simulink model "NeuronalNetwork"  (R2019b)
settings: Solver=VariableStepAuto  StartTime=0.0  StopTime=10.0  RelTol=1e-3
libraries: neural x1006
(part 3 of 11)

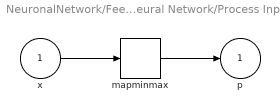
== system NeuronalNetwork/Feed-Forward Neural Network/Process Input 1 ==
  x : Inport  PortDimensions=1001  SampleTime=0.1
      mask Display: e = 0.06;c1 = [120 230 180]/255;c2 = ([120 230 180]+0)/(256+128);c3 = ([120 230 180]+128)/(256+128);patch([0 1 1 0],[0 0 1 1],c1);patch([0 1 1 1-e 1-e 0+e],[0 0 1 1-e 0+e 0+e],c2);patch([0 0 1 1-e 0+e 0+e],[0 1 1 1-e 1-e 0+e],c3);plot([0 1 1 0 0],[0 0 1 1 0]);
  mapminmax : neural/Processing Functions/mapminmax  xmin=[0.785398163397448278999490867136;0.709441408668645134838470767136;0.654230142742192599669692754105;0.615290765915770587746180808608;0.587466151596020225156280503143;0.565842136942244167130411369726;0.546291593455738633267060322396;0.525717673015665631908177601872;0.502090498167535370654945836577;0.474356865564650509448085813347;0.442284345023452152290133199131;0.406280540041972670906034181826;0.367209347491981086264445366396;0.326214334745977607710187839984;0.284555939084002673666873306502;0.243470447246644017269545656745;0.204059640191000424280787228781;0.167217606121480955039260152262;0.133595803186941530782405607169;0.10360143396444709829040675686;0.0774200746013615770380056346767;0.0550523483133633639852178021101;0.0363557636519837856781123264227;0.0210854164112119768503816885641;0.00892993062022617856143824610626;-0.000458871247863035236491668911185;-0.00744270835532989671889936289517;-0.0123794028861010652065033355029;-0.015610386427028499767288849398;-0.0174522405278876302503476836137;-0.0181914442101640538851370365592;-0.0180816228653828403594161500223;-0.0173427132861856403422962102923;-0.0161615638120036209102181601338;-0.014693574671496234529399771418;-0.0130650544686303771158009112696;-0.011376028220230871568219299661;-0.00970328347784943368026233656565;-0.00810348577435582306804917607224;-0.00661623389916599080606829375029;-0.00526695972456092675884065101855;-0.00406960663466815475430848891847;-0.00302904517984270427177762030624;-0.0021432046089739920091687963577;-0.00140491475077597627318937156815;-0.000803464748226234704020498611499;-0.00032589388241399674939202668611;4.19643425959570492977945832536e-05;0.000314660051512039018462019157596;0.000506500199471515699656265496742;0.000631090187944938207920131389983;0.000701017687264604560937186761294;0.000727653958252361121594731230289;0.000721049983764654456308562657796;0.000689907050786198183800479455385;0.000641603900344955846435368584935;0.000582265058452824391110880242195;0.000516857380913116060128231765702;0.000449304119792381939646475075278;0.000382607903842702157248822913971;0.000318975892022121954028079926502;0.00025994199600432033037122891983;0.000206482473331437432761958916672;0.000159122375285702943870091985445;0.000118031306518329159871427691542;8.31077348832920392851519864053e-05;5.4051700136836799970296851825e-05;3.04262305537150723466766066849e-05;1.17081084609615970748563995585e-05;-2.67115014418450869015941862017e-06;-1.32931011052050962462089955807e-05;-2.07278972408353467926644952968e-05;-2.5516458101115802037384128198e-05;-2.81582413605985237836648593657e-05;-2.91036346533601886221731547266e-05;-2.87500683957553349046065704897e-05;-2.7441043791043284727493301034e-05;-2.5467369312748289189585193526e-05;-2.30699985457327727544907247648e-05;-2.04439585727023143135738791898e-05;-1.77429484629065825629368191585e-05;-1.50842700734621359970333287492e-05;-1.25538272714997845014295307919e-05;-1.02109943727057839168992359191e-05;-8.09321005279528549181122798473e-06;-6.22019955787145306658203480765e-06;-4.5977662959106879725368344225e-06;-3.22112454465006692316819680855e-06;-2.07776889160626865304948296398e-06;-1.14989399091491861781832994893e-06;-4.16391101376589745086675975472e-07;1.45543456175900587368232663721e-07;5.59147637080315007551689632237e-07;8.47138112325396264168375637382e-07;1.03101689918894123820791719481e-06;1.13059865269882209304341813549e-06;1.16371964531403193632286274806e-06;1.1460927618056615528985275887e-06;1.09127662106800471519818529487e-06;1.01073089342484934149979380891e-06;9.13933864143956498082843609154e-07;8.08542119923316704444005154073e-07;7.00575833345595810897066257894e-07;5.94616389681945634038129355758e-07;4.94006026530158237619616556913e-07;4.01041718500749766462831757963e-07;3.17157717200089450670930091292e-07;2.43092999285821065313939470798e-07;1.79041373282728955018683336675e-07;1.24783202215539290591550525278e-07;7.97986305922648853083956055343e-08;4.33629090412779305552248843014e-08 ...(+32708 chars)]  xmax=[2.82842712474619029094924371748;2.6907248094147417916133235849;2.58020759331951055060017097276;2.50395147717411070686921448214;2.46533424855868155134430708131;2.46551192777841432501872986904;2.50454790897430124019251707068;2.58213929858001245420950908738;2.69802941507372606722015007108;2.85220466520313253866447666951;3.04495563555447468218062567757;3.27686722507688932282121641038;3.54879026713434519990642002085;3.86183244474606901519564416958;4.21738820750680876159321996965;4.61720859580680187406187542365;5.06349713639733156611555386917;5.55901129811952188219947856851;6.10715116028912508028270167415;6.71202505509323366084117878927;7.37849136369341529473331320332;8.11218263018648677586952544516;8.91952127514631776250553230057;9.80773602729153459733879572013;10.7848862060082755220946637564;11.8598985203906295282649807632;13.0426189082958980947068994283;14.3438804207005610180658550235;15.7755872534637600068663232378;17.350814607789420307426553336;19.0839239744165602985503937816;20.9906935650539203663811349543;23.0884638725804478553982335143;25.3962986713378917613681551302;27.9351621315887186369764094707;30.7281130918045413125128106913;33.8005178921375701861506968271;37.1802835129964748261954810005;40.898113081177228878004825674;44.9877861046339759809598035645;49.4864660815803105720078747254;54.4350384084046226007558288984;59.8784817931998247786395950243;65.8662766770315073472374933772;72.4528544823670870300702517852;79.6980918554584718549449462444;87.6678544540282871366798644885;96.434595259566734171130519826;106.07801287040436477582261432;116.685775762532813359939609654;128.354319094762757913485984318;141.189721288183704928087536246;155.308668332283758672929252498;170.839514567284055601703585126;187.923449570707646216760622337;206.715781743228035338688641787;227.387350252644409920321777463;250.126078164648419033255777322;275.138680875222235044930130243;302.65254537355946240495541133;332.917797419111877843533875421;366.209575425867228659626562148;402.83053172685879417258547619;443.113583959350023633305681869;487.424941585029387169925030321;536.167435060641309974016621709;589.784177925591166058438830078;648.762595099271493381820619106;713.638854009722308546770364046;785.00273883705028765689348802;863.503012183115743027883581817;949.853312909956798648636322469;1044.83864376355836611764971167;1149.3225077611828055523801595;1264.25475821829468259238637984;1390.68023377874555990274529904;1529.74825694829428357479628175;1682.72308248160311450192239136;1850.99539060791994415922090411;2036.09492957922134337422903627;2239.70442247302617033710703254;2463.67486467531898597371764481;2710.04235111161642635124735534;2981.04658620100281041231937706;3279.15124480546819540904834867;3607.06636927410909265745431185;3967.77300619170136997126974165;4364.55030680211802973644807935;4801.00533747408462659223005176;5281.10587121352637041127309203;5809.21645832716512813931331038;6390.13810415251191443530842662;7029.15191456086813559522852302;7732.0671060106651566457003355;8505.27381660614628344774246216;9355.80119826193731569219380617;10291.3813180840734275989234447;11320.5194498891632974846288562;12452.5713948754419106990098953;13697.8285343609477422432973981;15067.6113877955067437142133713;16574.3725265739303722511976957;18231.8097792305161419790238142;20054.990757153005688451230526;22060.4898328679119003936648369;24266.5388161544324248097836971;26693.192697769678488839417696;29362.5119675464957254007458687;32298.763164301020879065617919;35528.6394807310134638100862503;39081.5034288040042156353592873;42989.6537716843013186007738113;47288.6191488526383182033896446;52017.4810637378031970001757145;57219.2291701114882016554474831;62941.1520871225584414787590504;69235.2672958347393432632088661;76158.7940254181594355031847954;83774.673427959933178499341011;92152.1407707558828406035900116;101367.354847831433289684355259;111504.090332614548970013856888;122654.499365875992225483059883;134919.949302463588537648320198;148411.944232709938660264015198 ...(+25333 chars)]  ymin=-1  ymax=1
      settings: SourceProductName=Deep Learning Toolbox
  p : Outport  PortDimensions=1001  SampleTime=0.1
      mask Display: e = 0.06;c1 = [120 230 180]/255;c2 = ([120 230 180]+0)/(256+128);c3 = ([120 230 180]+128)/(256+128);patch([0 1 1 0],[0 0 1 1],c1);patch([0 1 1 1-e 1-e 0+e],[0 0 1 1-e 0+e 0+e],c2);patch([0 0 1 1-e 0+e 0+e],[0 1 1 1-e 1-e 0+e],c3);plot([0 1 1 0 0],[0 0 1 1 0]);
  wires:
  x/1 -> mapminmax/1
  mapminmax/1 -> p/1
